simulink model "sistema_1"  (R2025b)
settings: Solver=ode23t  StartTime=0.0  StopTime=10.0  MaxStep=1E-3  RelTol=1e-3
libraries: slpidlib x1, simulink x1
settings DataIOCC: ReturnWorkspaceOutputs=off  TimeSaveName=t
settings DebuggingCC: AlgebraicLoopMsg=none  ArtificialAlgebraicLoopMsg=none  MaxConsecutiveZCsMsg=none

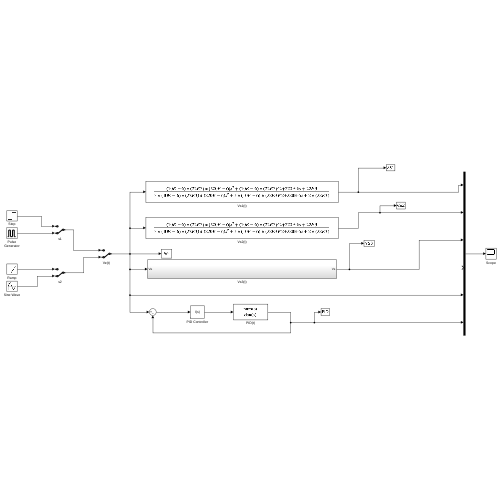
[thumbnail: Simulink's stored preview of the top-level diagram]
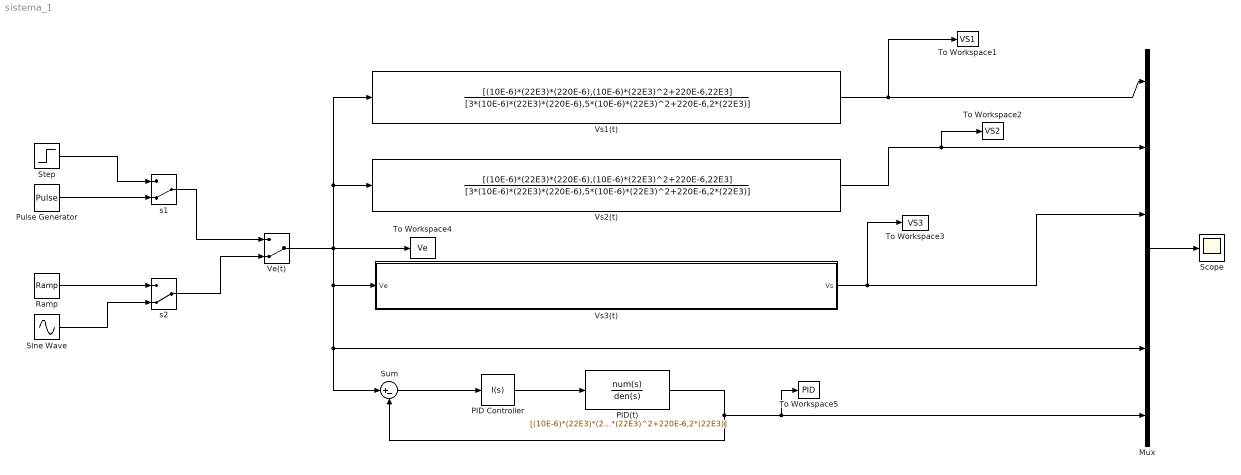
== system sistema_1 ==
  Mux : Mux  Inputs=6
  PID Controller : slpidlib/PID Controller  Controller=I  Form=Parallel  TimeDomain=Continuous-time  UseExternalTs=off  SampleTime=-1  IntegratorMethod=Forward Euler  FilterMethod=Forward Euler  ControllerParametersSource=internal  P=168.0717421143  I=6547.87290036297  UseKiTs=off  D=0.386154983035383  UseExternalDerivativeSource=off  N=291.659819026815  UseFilter=on  TunerSelectOption=Transfer Function Based (PID Tuner App)  InitialConditionSource=internal  InitialConditionForIntegrator=0  InitialConditionForFilter=0  DifferentiatorICPrevScaledInput=0  ExternalReset=none  TrackingMode=off  Kt=1  LimitOutput=off  SatLimitsSource=internal  UpperSaturationLimit=inf  LowerSaturationLimit=-inf  LinearizeAsGain=on  AntiWindupMode=none  Kb=1  LimitIntegrator=off  UpperIntegratorSaturationLimit=inf  LowerIntegratorSaturationLimit=-inf  POutMin=[]  POutMax=[]  IOutMin=[]  IOutMax=[]  DOutMin=[]  DOutMax=[]  NOutMin=[]  NOutMax=[]  SumOutMin=[]  SumOutMax=[]  SaturationOutMin=[]  SaturationOutMax=[]  PParamMin=[]  PParamMax=[]  IParamMin=[]  IParamMax=[]  DParamMin=[]  DParamMax=[]  NParamMin=[]  NParamMax=[]  KbParamMin=[]  KbParamMax=[]  KtParamMin=[]  KtParamMax=[]  KbOutMin=[]  KbOutMax=[]  KtOutMin=[]  KtOutMax=[]  IntegratorOutMin=[]  IntegratorOutMax=[]  FilterOutMin=[]  FilterOutMax=[]  SumI1OutMin=[]  SumI1OutMax=[]  SumI2OutMin=[]  SumI2OutMax=[]  SumI3OutMin=[]  SumI3OutMax=[]  SumI4OutMin=[]  SumI4OutMax=[]  SumDOutMin=[]  SumDOutMax=[]  DifferentiatorOutMin=[]  DifferentiatorOutMax=[]  FilterDiffOutCoefMin=[]  FilterDiffOutCoefMax=[]  ReciprocalOutMin=[]  ReciprocalOutMax=[]  SumDenOutMin=[]  SumDenOutMax=[]  SumNumOutMin=[]  SumNumOutMax=[]  DivideOutMin=[]  DivideOutMax=[]  UdiffTsProdOutMin=[]  UdiffTsProdOutMax=[]  NTsProdOutMin=[]  NTsProdOutMax=[]  UintegralTsProdOutMin=[]  UintegralTsProdOutMax=[]  UngainTsProdOutMin=[]  UngainTsProdOutMax=[]  ClampingZeroOutDataTypeStr=Inherit: Inherit via back propagation  ClampingZeroOutMin=[]  ClampingZeroOutMax=[]  FilterDenConstantOutDataTypeStr=Inherit: Inherit via back propagation  FilterDenConstantOutMin=[]  FilterDenConstantOutMax=[]  PCopyOutDataTypeStr=Inherit: Inherit via back propagation  PCopyOutMin=[]  PCopyOutMax=[]  NCopyOutDataTypeStr=Inherit: Inherit via back propagation  NCopyOutMin=[]  NCopyOutMax=[]  IntegratorContinuousStateAttributes=''  IntegratorStateMustResolveToSignalObject=off  IntegratorRTWStateStorageClass=Auto  FilterContinuousStateAttributes=''  FilterStateMustResolveToSignalObject=off  FilterRTWStateStorageClass=Auto  ParallelPVariant=Disabled  IdealPVariant=Disabled  IVariant=InternalParameters  DVariant=Disabled  IntegratorVariant=Continuous  SatVariant=Disabled  AWVariant=Passthrough  PCopyVariant=Disabled  TRVariant=Disabled  FdbkBlocksVariant=Forward  IdealPFdbkVariant=Disabled  SatFdbkVariant=Disabled  DerivativeFilterVariant=Disabled  NVariant=Disabled  NCopyVariant=Disabled_SignalSpec  FilterICVariant=Disabled  IntegratorICVariant=InternalICs  ExternalResetVariant=Disabled  TRSumVariant=Passthrough  SumFdbkVariant=Disabled  SumVariant=Passthrough_I  TsampFilterVariant=InternalTs  TsampNgainVariant=Passthrough  TsampIntegralVariant=Disabled_SignalSpec  ExternalSaturationOutDataTypeStr=Inherit: Same as second input  DerivativeSourceVariant=Disabled  PreIntVariant=InternalPreInt
  PID(t) : TransferFcn  Numerator=[(10E-6)*(22E3)*(220E-6),(10E-6)*(22E3)^2+220E-6,22E3]  Denominator=[3*(10E-6)*(22E3)*(220E-6),5*(10E-6)*(22E3)^2+220E-6,2*(22E3)]
  Pulse Generator : DiscretePulseGenerator  PulseType=Time based  Period=10  PulseWidth=10  PhaseDelay=1
  Ramp : simulink/Sources/Ramp  slope=1/10  start=0  InitialOutput=0
  Scope : Scope
      settings: ActiveDisplayYMinimum=-0.80012791908363812  ActiveDisplayYMaximum=1.6998720809163623
  Sine Wave : Sin  Frequency=pi/2  SampleTime=0
  Step : Step  Time=0  SampleTime=0.001
  Sum : Sum  Inputs=|+-
  To Workspace1 : ToWorkspace  VariableName=VS1  SampleTime=-1
  To Workspace2 : ToWorkspace  VariableName=VS2  SampleTime=-1
  To Workspace3 : ToWorkspace  VariableName=VS3  SampleTime=-1
  To Workspace4 : ToWorkspace  VariableName=Ve  SampleTime=-1
  To Workspace5 : ToWorkspace  VariableName=PID  SampleTime=-1
  Ve(t) : ManualSwitch  CurrentSetting=0
  Vs1(t) : TransferFcn  Numerator=[(10E-6)*(22E3)*(220E-6),(10E-6)*(22E3)^2+220E-6,22E3]  Denominator=[3*(10E-6)*(22E3)*(220E-6),5*(10E-6)*(22E3)^2+220E-6,2*(22E3)]
  Vs2(t) : TransferFcn  Numerator=[(10E-6)*(22E3)*(220E-6),(10E-6)*(22E3)^2+220E-6,22E3]  Denominator=[3*(10E-6)*(22E3)*(220E-6),5*(10E-6)*(22E3)^2+220E-6,2*(22E3)]
  Vs3(t) : Subsystem
  s1 : ManualSwitch  CurrentSetting=0
  s2 : ManualSwitch  CurrentSetting=0
  wires:
  Mux/1 -> Scope/1
  s1/1 -> Ve(t)/1
  Ve(t)/1 -> Vs1(t)/1, Vs2(t)/1, To Workspace4/1, Sum/1, Mux/5, Vs3(t)/1(Ve)
  Vs2(t)/1 -> To Workspace2/1, Mux/2
  Vs1(t)/1 -> To Workspace1/1, Mux/1
  Step/1 -> s1/1
  Pulse Generator/1 -> s1/2
  Sine Wave/1 -> s2/2
  Ramp/1 -> s2/1
  s2/1 -> Ve(t)/2
  Sum/1 -> PID Controller/1
  Vs3(t)/1(Vs) -> Mux/3, To Workspace3/1
  PID Controller/1 -> PID(t)/1
  PID(t)/1 -> Sum/2, To Workspace5/1, Mux/6

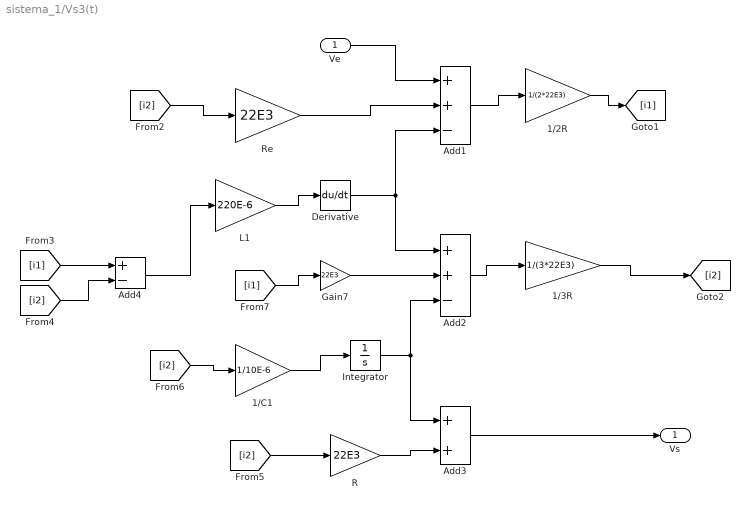
== system sistema_1/Vs3(t) ==
  Ve : Inport
  1/2R : Gain  Gain=1/(2*22E3)
  1/3R : Gain  Gain=1/(3*22E3)
  1/C1 : Gain  Gain=1/10E-6
  Add1 : Sum  Inputs=++-
  Add2 : Sum  Inputs=++-
  Add3 : Sum
  Add4 : Sum  Inputs=+-
  Derivative : Derivative
  Gain7 : Gain  Gain=22E3
  Integrator : Integrator
  L1 : Gain  Gain=220E-6
  R : Gain  Gain=22E3
  Re : Gain  Gain=22E3
  Vs : Outport
  wires:
  Integrator/1 -> Add3/1, Add2/3
  Add3/1 -> Vs/1
  [i1] -> Gain7/1
  Add2/1 -> 1/3R/1
  Add4/1 -> L1/1
  [i2] -> Add4/2
  1/2R/1 -> [i1]
  1/3R/1 -> [i2]
  Gain7/1 -> Add2/2
  [i2] -> 1/C1/1
  [i2] -> R/1
  1/C1/1 -> Integrator/1
  L1/1 -> Derivative/1
  Add1/1 -> 1/2R/1
  Ve/1 -> Add1/1
  Re/1 -> Add1/2
  [i1] -> Add4/1
  R/1 -> Add3/2
  Derivative/1 -> Add2/1, Add1/3
  [i2] -> Re/1
